simulink model "Quanser_Simulation"  (Simulink 9.0)
settings: Solver=ode1  StartTime=0.0  StopTime=40  FixedStep=0.002  RelTol=1e-3  EnableMultiTasking=on
values from neighbouring files (symbols this model uses):
  A = [0,1,0,0,0,0;0,0,0,0,0,0;0,0,0,1,0,0;0,0,0,0,0,0;0,0,0,0,0,1;0,0,0,0,0,0]    [ProportionalController.m]    (also in SecondOrderResponse.m = (log(PO/100))^2)
  B = [0,0,0;(1/Ix),0,0;0,0,0;0,(1/Iy),0;0,0,0;0,0,(1/Iz)]    [ProportionalController.m]
  C = [1,0,0,0,0,0;0,1,0,0,0,0;0,0,1,0,0,0]    [ProportionalController.m]
  D = [0,0,0;0,0,0;0,0,0]    [ProportionalController.m]
  K = [Ky(:,1),Kp(:,1),Kr(:,1),Ky(:,2),Kp(:,2),Kr(:,2)]    [ProportionalController.m]    (also in RLS_demo_init.m = 1; discrete1.m = 0.001; proportionalTest.m = [2.5273 0.4416 0 0 0 0)
  K_AMP = 3    [ProportionalController.m]
  V_bias = 2    [ProportionalController.m]
  VMAX_AMP = 24    [ProportionalController.m]
  VMAX_DAC = 10    [ProportionalController.m]
libraries: simulink_extras x5
settings Model: SuppressorTable=22 serialization::archive 11 0 6 0 0 0 0 0  Creator=hpineros  LastModifiedBy=YvesDaoud  ExtModeTrigDuration=10000
settings SolverCC: PositivePriorityOrder=on
settings DataIOCC: LimitDataPoints=on  SignalLoggingSaveFormat=ModelDataLogs
settings OptimizationCC: ExpressionDepthLimit=2147483647  InitFltsAndDblsToZero=on
settings DebuggingCC: SaveWithParameterizedLinksMsg=none  SolverPrmCheckMsg=warning  FcnCallInpInsideContextMsg=warning  AllowSymbolicDim=off  StateNameClashWarn=warning  StrictBusMsg=Warning
settings RTWCC: SystemTargetFile=quarc_windows.tlc  TemplateMakefile=quarc_default_tmf  Description=QuaRC Win32 Target
settings STFCustomTargetCC: TargetFcnLib=ansi_tfl_tmw.mat  TargetPreCompLibLocation=C:\PROGRA~3\QUARC\lib\2015b\windows\release  GeneratePreprocessorConditionals=Disable all  CPPClassGenCompliant=on  SystemTargetFile=quarc_windows.tlc
settings GRTTargetCC: TargetFcnLib=ansi_tfl_tmw.mat  TargetPreCompLibLocation=C:\PROGRA~3\QUARC\lib\2015b\windows\release  ParMdlRefBuildCompliant=off  CompOptLevelCompliant=off  ConcurrentExecutionCompliant=off  GeneratePreprocessorConditionals=Disable all  CombineOutputUpdateFcns=off  MatFileLogging=off  GRTInterface=on  UseToolchainInfoCompliant=off  ExtMode=on  ExtModeMexFile=quarc_comm

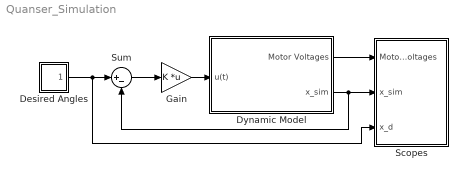
== system Quanser_Simulation ==
  Desired Angles : Subsystem
  Dynamic Model : Subsystem
  Gain : Gain  Gain=K  Multiplication=Matrix(K*u)
  Scopes : Subsystem
  Sum : Sum  Inputs=|+-
  wires:
  Desired Angles/1(x_d) -> Scopes/3(x_d), Sum/1
  Dynamic Model/1(Motor Voltages) -> Scopes/1(Motor Voltages)
  Dynamic Model/2(x_sim) -> Sum/2, Scopes/2(x_sim)
  Sum/1 -> Gain/1
  Gain/1 -> Dynamic Model/1(u(t))

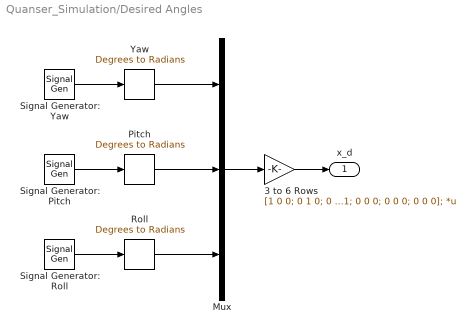
== system Quanser_Simulation/Desired Angles ==
  3 to 6 Rows : Gain  Gain=[1 0 0; 0 1 0; 0 0 1; 0 0 0; 0 0 0; 0 0 0];  Multiplication=Matrix(K*u)
  Mux : Mux  Inputs=3
  Pitch : simulink_extras/Transformations/Degrees to Radians
  Roll : simulink_extras/Transformations/Degrees to Radians
  Signal Generator: Pitch : SignalGenerator  WaveForm=square  Amplitude=5  Frequency=0.04
  Signal Generator: Roll : SignalGenerator  WaveForm=square  Amplitude=5  Frequency=0.04
  Signal Generator: Yaw : SignalGenerator  WaveForm=square  Amplitude=5  Frequency=0.04
  Yaw : simulink_extras/Transformations/Degrees to Radians
  x_d : Outport
  wires:
  3 to 6 Rows/1 -> x_d/1
  Mux/1 -> 3 to 6 Rows/1
  Roll/1 -> Mux/3
  Pitch/1 -> Mux/2
  Yaw/1 -> Mux/1
  Signal Generator: Roll/1 -> Roll/1
  Signal Generator: Pitch/1 -> Pitch/1
  Signal Generator: Yaw/1 -> Yaw/1

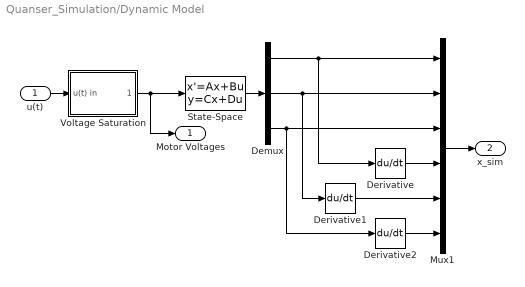
== system Quanser_Simulation/Dynamic Model ==
  u(t) : Inport
  Demux : Demux  Outputs=3
  Derivative : Derivative
  Derivative1 : Derivative
  Derivative2 : Derivative
  Mux1 : Mux  Inputs=6
  State-Space : StateSpace  A=A  B=B  C=C  D=D  InitialCondition=0
  Voltage Saturation : Subsystem
  Motor Voltages : Outport
  x_sim : Outport  Port=2
  wires:
  Derivative2/1 -> Mux1/6
  Derivative1/1 -> Mux1/5
  Derivative/1 -> Mux1/4
  State-Space/1 -> Demux/1
  Mux1/1 -> x_sim/1
  Voltage Saturation/1(u(t) out) -> Motor Voltages/1, State-Space/1
  u(t)/1 -> Voltage Saturation/1(u(t) in)
  Demux/1 -> Mux1/1, Derivative/1
  Demux/2 -> Derivative1/1, Mux1/2
  Demux/3 -> Derivative2/1, Mux1/3

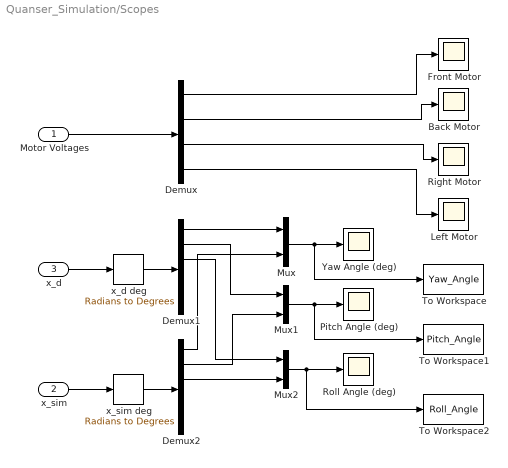
== system Quanser_Simulation/Scopes ==
  Motor Voltages : Inport
  x_sim : Inport  Port=2
  x_d : Inport  Port=3
  Back Motor : Scope
  Demux : Demux
  Demux1 : Demux  Outputs=6
  Demux2 : Demux  Outputs=6
  Front Motor : Scope
  Left Motor : Scope
  Mux : Mux  Inputs=2
  Mux1 : Mux  Inputs=2
  Mux2 : Mux  Inputs=2
  Pitch Angle (deg) : Scope
  Right Motor : Scope
  Roll Angle (deg) : Scope
  To Workspace : ToWorkspace  VariableName=Yaw_Angle  SaveFormat=Timeseries  SampleTime=-1
      settings: Save2DSignal=2-D array (concatenate along first dimension)
  To Workspace1 : ToWorkspace  VariableName=Pitch_Angle  SaveFormat=Timeseries  SampleTime=-1
      settings: Save2DSignal=2-D array (concatenate along first dimension)
  To Workspace2 : ToWorkspace  VariableName=Roll_Angle  SaveFormat=Timeseries  SampleTime=-1
      settings: Save2DSignal=2-D array (concatenate along first dimension)
  Yaw Angle (deg) : Scope
  x_d deg : simulink_extras/Transformations/Radians to Degrees
  x_sim deg : simulink_extras/Transformations/Radians to Degrees
  wires:
  Mux2/1 -> To Workspace2/1, Roll Angle (deg)/1
  Mux1/1 -> To Workspace1/1, Pitch Angle (deg)/1
  Mux/1 -> Yaw Angle (deg)/1, To Workspace/1
  x_sim/1 -> x_sim deg/1
  x_d/1 -> x_d deg/1
  Motor Voltages/1 -> Demux/1
  Demux/1 -> Front Motor/1
  Demux/2 -> Back Motor/1
  Demux/3 -> Right Motor/1
  Demux/4 -> Left Motor/1
  x_d deg/1 -> Demux1/1
  Demux1/1 -> Mux/1
  Demux1/2 -> Mux1/1
  Demux1/3 -> Mux2/1
  Demux2/1 -> Mux/2
  Demux2/2 -> Mux1/2
  Demux2/3 -> Mux2/2
  x_sim deg/1 -> Demux2/1

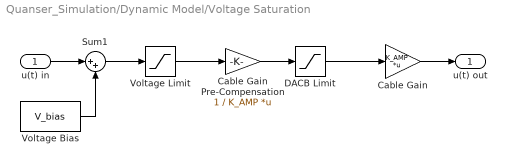
== system Quanser_Simulation/Dynamic Model/Voltage Saturation ==
  u(t) in : Inport
  Cable Gain : Gain  Gain=K_AMP  Multiplication=Matrix(K*u)  SaturateOnIntegerOverflow=on  OutDataTypeStr=Inherit: Same as input  ParamDataTypeStr=Inherit: Same as input
  Cable Gain Pre-Compensation : Gain  Gain=1 / K_AMP  Multiplication=Matrix(K*u)  SaturateOnIntegerOverflow=on  OutDataTypeStr=Inherit: Same as input  ParamDataTypeStr=Inherit: Same as input
  DACB Limit : Saturate  UpperLimit=VMAX_DAC  LowerLimit=-VMAX_DAC
  Sum1 : Sum  Inputs=|++
  Voltage Bias : Constant  Value=V_bias
  Voltage Limit : Saturate  UpperLimit=VMAX_AMP  LowerLimit=0
  u(t) out : Outport
  wires:
  Cable Gain Pre-Compensation/1 -> DACB Limit/1
  DACB Limit/1 -> Cable Gain/1
  Cable Gain/1 -> u(t) out/1
  Voltage Limit/1 -> Cable Gain Pre-Compensation/1
  Voltage Bias/1 -> Sum1/2
  u(t) in/1 -> Sum1/1
  Sum1/1 -> Voltage Limit/1
